simulink model "dvfs_systolic_model"  (R2025b)
settings: Solver=VariableStepAuto  StartTime=0.0  StopTime=10.0  RelTol=1e-3
settings Model: Creator=Pramod Kumar Singh  LastModifiedBy=Pramod Kumar Singh

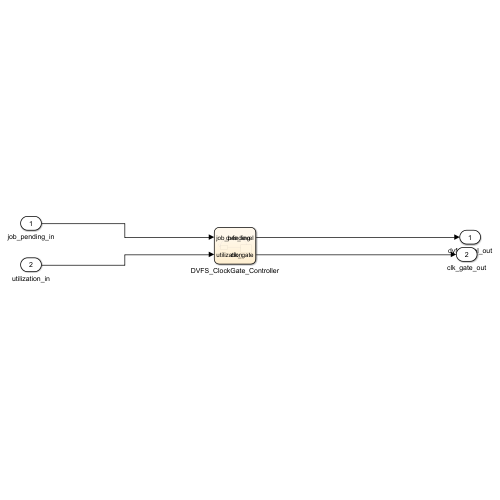
[thumbnail: Simulink's stored preview of the top-level diagram]
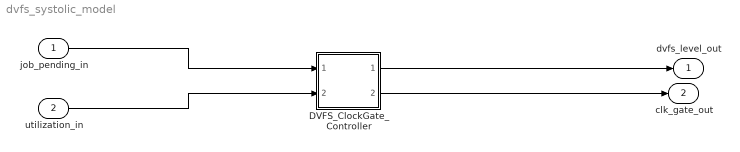
== system dvfs_systolic_model ==
  job_pending_in : Inport
  utilization_in : Inport  Port=2
  DVFS_ClockGate_Controller : Stateflow chart  TreatAsAtomicUnit=on
  dvfs_level_out : Outport
  clk_gate_out : Outport  Port=2
  wires:
  job_pending_in/1 -> DVFS_ClockGate_Controller/1(job_pending)
  utilization_in/1 -> DVFS_ClockGate_Controller/2(utilization)
  DVFS_ClockGate_Controller/1(dvfs_level) -> dvfs_level_out/1
  DVFS_ClockGate_Controller/2(clk_gate) -> clk_gate_out/1

== stateflow chart dvfs_systolic_model/DVFS_ClockGate_Controller ==
  state ACTIVE
    entry: clk_gate = false;
    during: if utilization > 0.8
    dvfs_level = 5;
    elseif utilization > 0.6
    dvfs_level = 4;
    elseif utilization > 0.4
    dvfs_level = 3;
    elseif utilization > 0.2
    dvfs_level = 2;
    else
    dvfs_level = 1;
    end
  state IDLE
    entry: dvfs_level = 1; clk_gate = true;
  ACTIVE -> IDLE : [job_pending == false]
  (default) -> IDLE
  IDLE -> ACTIVE : [job_pending == true]
  data: job_pending input boolean; utilization input double; dvfs_level output uint8; clk_gate output boolean
